simulink model "ex2"  (R2017b)
settings: Solver=VariableStepAuto  StartTime=0.0  StopTime=30.0  RelTol=1e-3
settings Model: Creator=User  LastModifiedBy=User

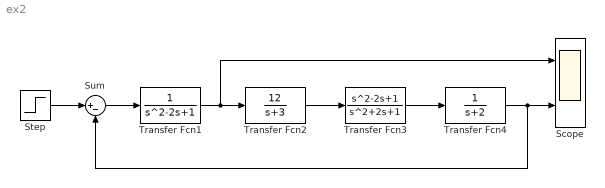
== system ex2 ==
  Scope : Scope  NumInputPorts=2
  Step : Step  Time=0  SampleTime=0
  Sum : Sum  Inputs=|+-
  Transfer Fcn1 : TransferFcn  Denominator=[1 -2 1]
  Transfer Fcn2 : TransferFcn  Numerator=[12]  Denominator=[1 3]
  Transfer Fcn3 : TransferFcn  Numerator=[1 -2 1]
  Transfer Fcn4 : TransferFcn  Denominator=[1 2]
  wires:
  Step/1 -> Sum/1
  Sum/1 -> Transfer Fcn1/1
  Transfer Fcn1/1 -> Transfer Fcn2/1, Scope/1
  Transfer Fcn2/1 -> Transfer Fcn3/1
  Transfer Fcn3/1 -> Transfer Fcn4/1
  Transfer Fcn4/1 -> Scope/2, Sum/2
